simulink model "Sistema_Seguimiento_Tipo1_Con_Planta_Tipo_0_Sin_Matrices"  (R2016a)
settings: Solver=VariableStepAuto  StartTime=0.0  StopTime=50  RelTol=1e-3
values from neighbouring files (symbols this model uses):
  K = acker(A, B ,PLC)    [Final_2017_Ejercicio_3.m]    (also in Final_2018_Ejercicio_1.m; Final_2018_Ejercicio_2.m = 10; Final_2019_Ejercicio_3.m = acker(Ahat, Bhat ,PLC2); Final_2020.m = acker(Ahat, Bhat ,PLC))
settings Model: Creator=Abel  LastModifiedBy=Abel

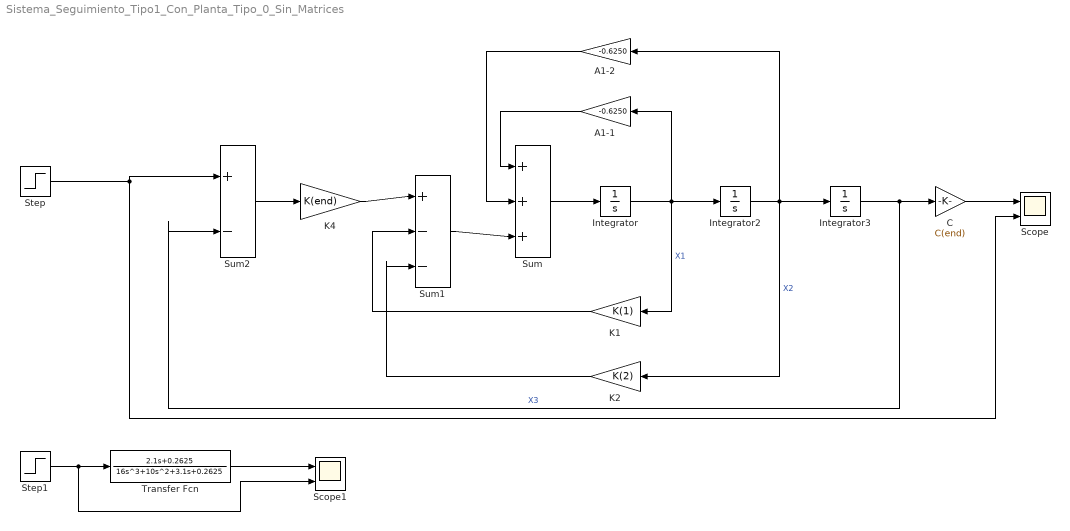
== system Sistema_Seguimiento_Tipo1_Con_Planta_Tipo_0_Sin_Matrices ==
  A1-1 : Gain  Gain=-0.6250
  A1-2 : Gain  Gain=-0.6250
  C : Gain  Gain=C(end)
  Integrator : Integrator
  Integrator2 : Integrator
  Integrator3 : Integrator
  K1 : Gain  Gain=K(1)
  K2 : Gain  Gain=K(2)
  K4 : Gain  Gain=K(end)
  Scope : Scope  NumInputPorts=2
  Scope1 : Scope  NumInputPorts=2
  Step : Step  SampleTime=0
  Step1 : Step  SampleTime=0
  Sum : Sum  Inputs=|+|+|+|
  Sum1 : Sum  Inputs=|+|-|-|
  Sum2 : Sum  Inputs=|+|-|
  Transfer Fcn : TransferFcn  Numerator=[2.1 0.2625]  Denominator=[16 10 3.1 0.2625]
  wires:
  Integrator/1 -> K1/1, A1-1/1, Integrator2/1  "X1"
  Sum/1 -> Integrator/1
  A1-1/1 -> Sum/1
  A1-2/1 -> Sum/2
  Integrator2/1 -> Integrator3/1, K2/1, A1-2/1  "X2"
  K2/1 -> Sum1/3
  Sum2/1 -> K4/1
  Step/1 -> Scope/2, Sum2/1
  Sum1/1 -> Sum/3
  K1/1 -> Sum1/2
  Integrator3/1 -> Sum2/2, C/1  "X3"
  K4/1 -> Sum1/1
  C/1 -> Scope/1
  Step1/1 -> Scope1/2, Transfer Fcn/1
  Transfer Fcn/1 -> Scope1/1
